simulink model "simulation model"  (R2022b)
settings: Solver=VariableStepAuto  StartTime=0.0  StopTime=2  RelTol=1e-3
undefined symbols (not defined in the file): a_prop, ACCtime, alfa, alfaPRO, Ba, Bf, Bp, Bv, IPR, matrixA, Ng_safe, No_perf, No_safe, Np, Np_safe, optimal_rotation, P3tDIVP2t_perf, P3tDIVP2t_safe, Q, Q_safe, T45_perf, T45_safe, Wf, xfuel, xlin, y, Yangle
libraries: fl_lib x31, nesl_utility x15, sh_lib x14, simulink x7, slpidlib x4, SimscapeFluids_lib x3
(part 1 of 2)
settings Model: PacingRate=10  Creator=48519  LastModifiedBy=48519
settings ModelReferenceCC: EnableRefExpFcnMdlSchedulingChecks=on

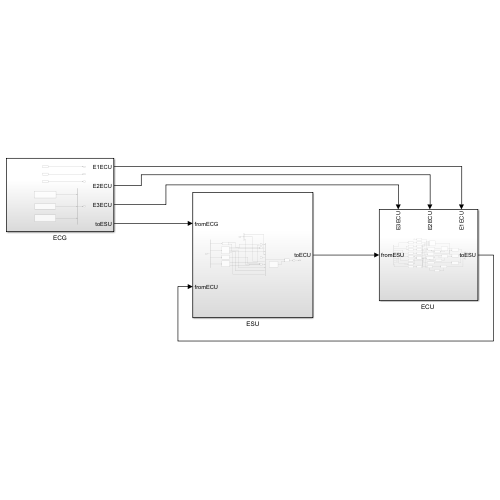
[thumbnail: Simulink's stored preview of the top-level diagram]
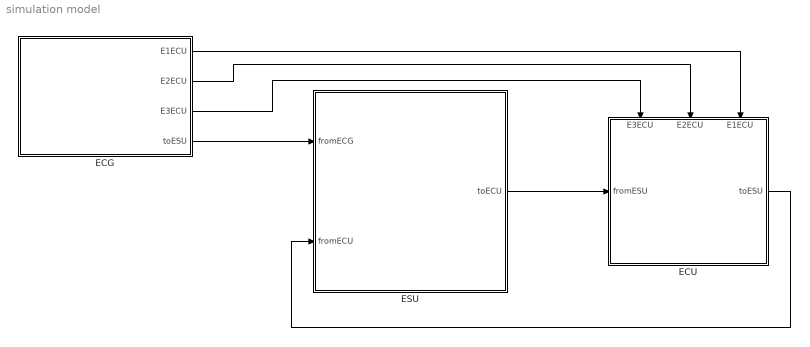
== system simulation model ==
  ECG : Subsystem
  "ECU " : Subsystem
      settings: PortSchema="{\"entries\":[{\"content\":{\"sides\":[{\"content\":{\"connectorIds\":[\"In1\"]},\"type\":\"ConnectorPlacement.EquallySpacedRectSide\",\"uuid\":\"8033a1fc-fa43-4d06-87e8-a4fef786c523\"},{\"content\":{\"connectorIds\":[\"Out1\"],\"side\":\"RIGHT\"},\"type\":\"ConnectorPlacement.EquallySpacedRectSide\",\"uuid\":\"5ca676c1-3d8d-4463-b14b-f5be12773dca\"},{\"content\":{\"connectorIds\":[\"In2\",\"In3\",\"In4\"],\"side\":\"TOP\"},\"type\":\"ConnectorPlacement.EquallySpacedRectSide\",\"uuid\":\"b18e2333-642d-4289-9df9-5f2a20e0ab9d\"}]},\"type\":\"ConnectorPlacement.EquallySpacedConnector\",\"uuid\":\"ecce7f03-20fc-4eea-af2c-957349ea8142\"}],\"packageUris\":[\"http://schema.mathworks.com/mf0/Connector/R2020b\"],\"version\":\"1.0\"}"
  ESU : Subsystem
  wires:
  ECG/4(toESU) -> ESU/1(fromECG)
  ESU/1(toECU) -> "ECU "/1(fromESU)
  "ECU "/1(toESU) -> ESU/2(fromECU)
  ECG/3(E3ECU) -> "ECU "/2(E3ECU)
  ECG/2(E2ECU) -> "ECU "/3(E2ECU)
  ECG/1(E1ECU) -> "ECU "/4(E1ECU)

== system simulation model/ECG ==
  Bus Creator : BusCreator  Inputs=4
  Emergency4 : Subsystem
  Emergency5 : Subsystem
  Emergency6 : Subsystem
  From Workspace : FromWorkspace  VariableName=Emerg3
  From Workspace1 : FromWorkspace  VariableName=Emerg1
  From Workspace2 : FromWorkspace  VariableName=Emerg2
  E1ECU : Outport
  E2ECU : Outport  Port=2
  E3ECU : Outport  Port=3
  toESU : Outport  Port=4
  wires:
  Emergency6/1(dP3e6) -> Bus Creator/4
  From Workspace1/1 -> E1ECU/1
  From Workspace/1 -> E3ECU/1
  From Workspace2/1 -> E2ECU/1
  Emergency4/1(dP2e4) -> Bus Creator/1
  Emergency5/2(dT1e5) -> Bus Creator/3
  Emergency5/1(dP0e5) -> Bus Creator/2
  Bus Creator/1 -> toESU/1

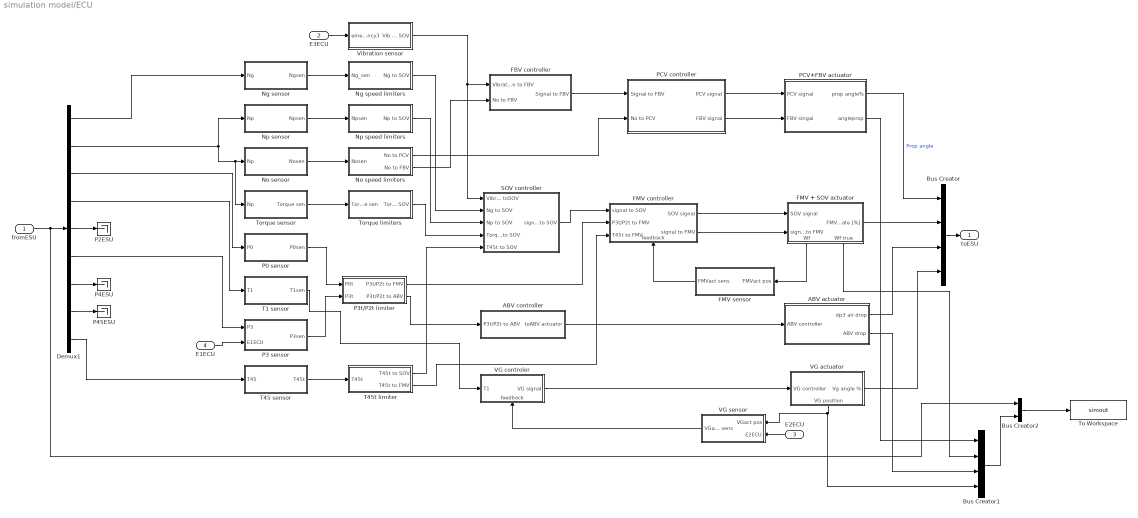
== system simulation model/ECU  ==
  fromESU : Inport
  E3ECU : Inport  Port=2
  E2ECU : Inport  Port=3
  E1ECU : Inport  Port=4
  " FMV controller" : Subsystem
      settings: PortSchema="{\"entries\":[{\"content\":{\"sides\":[{\"content\":{\"connectorIds\":[\"In1\",\"In2\",\"In3\"]},\"type\":\"ConnectorPlacement.EquallySpacedRectSide\",\"uuid\":\"38a2bfe9-8c47-42f1-bcd8-9832b9b327c4\"},{\"content\":{\"connectorIds\":[\"Out1\",\"Out2\"],\"side\":\"RIGHT\"},\"type\":\"ConnectorPlacement.EquallySpacedRectSide\",\"uuid\":\"0c090e16-2748-47be-b0e4-e5bed405b7d9\"},{\"content\":{\"connectorIds\":[],\"side\":\"TOP\"},\"type\":\"ConnectorPlacement.EquallySpacedRectSide\",\"uuid\":\"289f8d23-a454-4bfb-b029-d000a7415460\"},{\"content\":{\"connectorIds\":[\"In4\"],\"side\":\"BOTTOM\"},\"type\":\"ConnectorPlacement.EquallySpacedRectSide\",\"uuid\":\"f8021000-ba0a-47f6-928e-a2ead77e7ac1\"}]},\"type\":\"ConnectorPlacement.EquallySpacedConnector\",\"uuid\":\"1bac82f5-ade2-4038-9fa3-c74e21ed34d4\"}],\"packageUris\":[\"http://schema.mathworks.com/mf0/Connector/R2020b\"],\"version\":\"1.0\"}"
  ABV actuator : Subsystem
  ABV controller : Subsystem
  Bus Creator : BusCreator  Inputs=4
  Bus Creator1 : BusCreator  Inputs=4
  Bus Creator2 : BusCreator  Inputs=2
  Demux1 : Demux  Outputs=9
  FBV controller : Subsystem
  FMV + SOV actuator : Subsystem
      settings: PortSchema="{\"entries\":[{\"content\":{\"sides\":[{\"content\":{\"connectorIds\":[\"In1\",\"In2\"]},\"type\":\"ConnectorPlacement.EquallySpacedRectSide\",\"uuid\":\"38a2bfe9-8c47-42f1-bcd8-9832b9b327c4\"},{\"content\":{\"connectorIds\":[\"Out1\"],\"side\":\"RIGHT\"},\"type\":\"ConnectorPlacement.EquallySpacedRectSide\",\"uuid\":\"0c090e16-2748-47be-b0e4-e5bed405b7d9\"},{\"content\":{\"connectorIds\":[],\"side\":\"TOP\"},\"type\":\"ConnectorPlacement.EquallySpacedRectSide\",\"uuid\":\"289f8d23-a454-4bfb-b029-d000a7415460\"},{\"content\":{\"connectorIds\":[\"Out2\",\"Out3\"],\"side\":\"BOTTOM\"},\"type\":\"ConnectorPlacement.EquallySpacedRectSide\",\"uuid\":\"e366b5da-b3ec-4e5d-b0ef-8b87cef1eb6e\"}]},\"type\":\"ConnectorPlacement.EquallySpacedConnector\",\"uuid\":\"1bac82f5-ade2-4038-9fa3-c74e21ed34d4\"}],\"packageUris\":[\"http://schema.mathworks.com/mf0/Connector/R2020b\"],\"version\":\"1.0\"}"
  FMV sensor : Subsystem
  Ng sensor : Subsystem
  Ng speed limiters : Subsystem
  No sensor : Subsystem
  No speed limiters : Subsystem
  Np sensor : Subsystem
  Np speed limiters : Subsystem
  P0 sensor : Subsystem
  P2ESU : Terminator
  P3 sensor : Subsystem
  P3t/P2t limiter : Subsystem
  P45ESU : Terminator
  P4ESU : Terminator
  PCV controller : Subsystem
  PCV+FBV actuator : Subsystem
  SOV controller : Subsystem
  T1 sensor : Subsystem
  T45 sensor : Subsystem
  T45t limiter : Subsystem
  To Workspace : ToWorkspace  VariableName=simout  SaveFormat=Timeseries  SampleTime=-1
  Torque limiters : Subsystem
  Torque sensor : Subsystem
  VG actuator : Subsystem
      settings: PortSchema="{\"entries\":[{\"content\":{\"sides\":[{\"content\":{\"connectorIds\":[\"In1\"]},\"type\":\"ConnectorPlacement.EquallySpacedRectSide\",\"uuid\":\"39b00fd1-fd74-4dff-8589-67b80ee9d21f\"},{\"content\":{\"connectorIds\":[\"Out1\"],\"side\":\"RIGHT\"},\"type\":\"ConnectorPlacement.EquallySpacedRectSide\",\"uuid\":\"03fd2ba7-5317-42ec-98e7-2911bf7d9f9e\"},{\"content\":{\"connectorIds\":[],\"side\":\"TOP\"},\"type\":\"ConnectorPlacement.EquallySpacedRectSide\",\"uuid\":\"f7078396-c4bb-405d-aad9-135faa07c4e1\"},{\"content\":{\"connectorIds\":[\"Out2\"],\"side\":\"BOTTOM\"},\"type\":\"ConnectorPlacement.EquallySpacedRectSide\",\"uuid\":\"db5e57f9-c653-4944-8a82-ef51bf9c1c7f\"}]},\"type\":\"ConnectorPlacement.EquallySpacedConnector\",\"uuid\":\"a5cbbca1-7c96-4ab0-8754-d29e08537f1a\"}],\"packageUris\":[\"http://schema.mathworks.com/mf0/Connector/R2020b\"],\"version\":\"1.0\"}"
  VG controler : Subsystem
      settings: PortSchema="{\"entries\":[{\"content\":{\"sides\":[{\"content\":{\"connectorIds\":[\"In1\"]},\"type\":\"ConnectorPlacement.EquallySpacedRectSide\",\"uuid\":\"38a2bfe9-8c47-42f1-bcd8-9832b9b327c4\"},{\"content\":{\"connectorIds\":[\"Out1\"],\"side\":\"RIGHT\"},\"type\":\"ConnectorPlacement.EquallySpacedRectSide\",\"uuid\":\"0c090e16-2748-47be-b0e4-e5bed405b7d9\"},{\"content\":{\"connectorIds\":[],\"side\":\"TOP\"},\"type\":\"ConnectorPlacement.EquallySpacedRectSide\",\"uuid\":\"289f8d23-a454-4bfb-b029-d000a7415460\"},{\"content\":{\"connectorIds\":[\"In2\"],\"side\":\"BOTTOM\"},\"type\":\"ConnectorPlacement.EquallySpacedRectSide\",\"uuid\":\"9fd355d9-d690-4719-8550-140a79b88711\"}]},\"type\":\"ConnectorPlacement.EquallySpacedConnector\",\"uuid\":\"1bac82f5-ade2-4038-9fa3-c74e21ed34d4\"}],\"packageUris\":[\"http://schema.mathworks.com/mf0/Connector/R2020b\"],\"version\":\"1.0\"}"
  VG sensor : Subsystem
  Vibration sensor : Subsystem
  toESU : Outport
  wires:
  Ng sensor/1(Ngsen) -> Ng speed limiters/1(Ng_sen)
  Demux1/1 -> Ng sensor/1(Ng)
  Demux1/2 -> Np sensor/1(Np), Torque sensor/1(Np), No sensor/1(Np)
  fromESU/1 -> Bus Creator2/1, Demux1/1
  Demux1/3 -> P0 sensor/1(P0)
  Demux1/4 -> T1 sensor/1(T1)
  Demux1/5 -> P2ESU/1
  Demux1/6 -> P3 sensor/1(P3)
  Demux1/7 -> P4ESU/1
  Demux1/8 -> P45ESU/1
  Demux1/9 -> T45 sensor/1(T45)
  Np sensor/1(Npsen) -> Np speed limiters/1(Npsen)
  No sensor/1(Nosen) -> No speed limiters/1(Nosen)
  Torque sensor/1(Torque sen) -> Torque limiters/1(Torque sen)
  P3 sensor/1(P3sen) -> P3t/P2t limiter/2(P3t)
  P0 sensor/1(P0sen) -> P3t/P2t limiter/1(P0t)
  T45 sensor/1(T45t) -> T45t limiter/1(T45t)
  T45t limiter/2(T45t to FMV) -> " FMV controller"/3(T45t to FMV)
  P3t/P2t limiter/1(P3t/P2t to FMV) -> " FMV controller"/2(P3t/P2t to FMV)
  Ng speed limiters/1(Ng to SOV) -> SOV controller/2(Ng to SOV)
  Np speed limiters/1(Np to SOV) -> SOV controller/3(Np to SOV)
  " FMV controller"/2(signal to FMV) -> FMV + SOV actuator/2(signal to FMV)
  No speed limiters/1(No to PCV) -> PCV controller/2(No to PCV)
  No speed limiters/2(No to FBV) -> FBV controller/2(No to FBV)
  PCV controller/1(PCV signal) -> PCV+FBV actuator/1(PCV signal)
  Vibration sensor/1(Vib to SOV) -> FBV controller/1(Vibration to FBV), SOV controller/1(Vibration toSOV)
  T45t limiter/1(T45t to SOV) -> SOV controller/5(T45t to SOV)
  P3t/P2t limiter/2(P3t/P2t to ABV) -> ABV controller/1(P3t/P2t to ABV)
  PCV+FBV actuator/1(prop angle%) -> Bus Creator/1  "Prop angle"
  FMV + SOV actuator/1(FMV flow rate [%]) -> Bus Creator/2
  ABV actuator/1(dp3 air drop) -> Bus Creator/3
  VG actuator/1(Vg angle %) -> Bus Creator/4
  Bus Creator/1 -> toESU/1
  Torque limiters/1(Torque to SOV) -> SOV controller/4(Torque to SOV)
  E3ECU/1 -> Vibration sensor/1(emergency3)
  E1ECU/1 -> P3 sensor/2(E1ECU)
  E2ECU/1 -> VG sensor/2(E2ECU)
  FMV + SOV actuator/2(Wf) -> FMV sensor/1(FMVact pos)
  FMV sensor/1(FMVact sens) -> " FMV controller"/4(feedback)
  VG actuator/2(VG position) -> Bus Creator1/4, VG sensor/1(VGact pos)
  VG sensor/1(VGact sens) -> VG controler/2(feedback)
  PCV controller/2(FBV signal) -> PCV+FBV actuator/2(FBV singal)
  " FMV controller"/1(SOV signal) -> FMV + SOV actuator/1(SOV signal)
  T1 sensor/1(T1sen) -> VG controler/1(T1)
  Bus Creator1/1 -> Bus Creator2/2
  ABV actuator/2(ABV drop) -> Bus Creator1/3
  FMV + SOV actuator/3(Wf true) -> Bus Creator1/2
  PCV+FBV actuator/2(angleprop) -> Bus Creator1/1
  Bus Creator2/1 -> To Workspace/1
  FBV controller/1(Signal to FBV) -> PCV controller/1(Signal to FBV)
  SOV controller/1(signal to SOV) -> " FMV controller"/1(signal to SOV)
  ABV controller/1(toABV actuator) -> ABV actuator/1(ABV controller)
  VG controler/1(VG signal) -> VG actuator/1(VG controller)

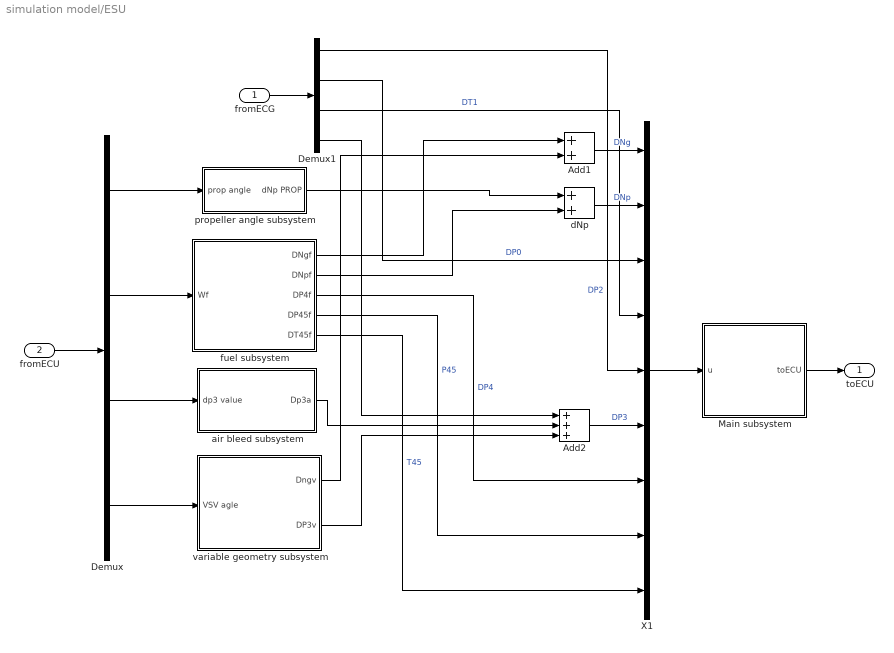
== system simulation model/ESU ==
  fromECG : Inport
  fromECU : Inport  Port=2
  Add1 : Sum
  Add2 : Sum  Inputs=+++
  Demux : Demux
  Demux1 : Demux
  Main subsystem : Subsystem
  X1 : BusCreator  Inputs=9
  air bleed subsystem : Subsystem
  dNp : Sum
  fuel subsystem : Subsystem
  propeller angle subsystem : Subsystem
  variable geometry subsystem : Subsystem
  toECU : Outport
  wires:
  fuel subsystem/2(DNpf) -> dNp/2
  fuel subsystem/3(DP4f) -> X1/7  "DP4"
  fuel subsystem/4(DP45f) -> X1/8  "P45"
  air bleed subsystem/1(Dp3a) -> Add2/2
  Demux/1 -> propeller angle subsystem/1(prop angle)
  Demux/4 -> variable geometry subsystem/1("VSV agle ")
  dNp/1 -> X1/2  "DNp"
  propeller angle subsystem/1(dNp PROP) -> dNp/1
  Add1/1 -> X1/1  "DNg"
  fuel subsystem/1(DNgf) -> Add1/1
  variable geometry subsystem/1(Dngv) -> Add1/2
  Demux1/1 -> X1/5  "DP2"
  Demux1/2 -> X1/3  "DP0"
  variable geometry subsystem/2(DP3v) -> Add2/3
  Add2/1 -> X1/6  "DP3"
  fuel subsystem/5(DT45f) -> X1/9  "T45"
  Demux1/3 -> X1/4  "DT1"
  Demux1/4 -> Add2/1
  X1/1 -> Main subsystem/1(u)
  Main subsystem/1(toECU) -> toECU/1
  fromECU/1 -> Demux/1
  Demux/3 -> air bleed subsystem/1(dp3 value)
  Demux/2 -> fuel subsystem/1(Wf)
  fromECG/1 -> Demux1/1

== system simulation model/ECG/Emergency4 ==
  Clock : Clock
  Clock1 : Clock
  Constant : Constant  Value=0
  Constant1 : Constant  Value=0
  From Workspace : FromWorkspace  VariableName=Emerg4
  Ramp : simulink/Sources/Ramp  slope=-0.07/450  start=ACCtime  InitialOutput=0
  Ramp1 : simulink/Sources/Ramp  slope=0.07/50  start=ACCtime+30  InitialOutput=0
  Switch : Switch  Criteria=u2 > Threshold  Threshold=ACCtime+40  SaturateOnIntegerOverflow=off  InputSameDT=off
  Switch1 : Switch  Criteria=u2 > Threshold  Threshold=ACCtime+30  SaturateOnIntegerOverflow=off  InputSameDT=off
  Switch2 : Switch  Criteria=u2 > Threshold  SaturateOnIntegerOverflow=off  InputSameDT=off
  dP2e4 : Outport
  wires:
  Ramp1/1 -> Switch1/1
  Ramp/1 -> Switch1/3
  Switch1/1 -> Switch/3
  Constant/1 -> Switch/1
  Clock/1 -> Switch/2
  Clock1/1 -> Switch1/2
  From Workspace/1 -> Switch2/2
  Constant1/1 -> Switch2/3
  Switch/1 -> Switch2/1
  Switch2/1 -> dP2e4/1

== system simulation model/ECG/Emergency5 ==
  Clock3 : Clock
  Constant1 : Constant  Value=0
  Constant2 : Constant  Value=0
  From Workspace : FromWorkspace  VariableName=Emerg5
  Ramp2 : simulink/Sources/Ramp  slope=-(0.05)/(300*300/2)  start=ACCtime  InitialOutput=0
  Switch2 : Switch  Criteria=u2 > Threshold  SaturateOnIntegerOverflow=off  InputSameDT=off
  Switch3 : Switch  Criteria=u2 > Threshold  Threshold=ACCtime+300  SaturateOnIntegerOverflow=off  InputSameDT=off
  dP0e5 : Outport
  dT1e5 : Outport  Port=2
  wires:
  Switch2/1 -> dT1e5/1, dP0e5/1
  Constant2/1 -> Switch3/1
  Ramp2/1 -> Switch3/3
  Clock3/1 -> Switch3/2
  Constant1/1 -> Switch2/3
  From Workspace/1 -> Switch2/2
  Switch3/1 -> Switch2/1

== system simulation model/ECG/Emergency6 ==
  Clock2 : Clock
  Constant1 : Constant  Value=0
  Constant2 : Constant  Value=0
  From Workspace : FromWorkspace  VariableName=Emerg6
  Ramp3 : simulink/Sources/Ramp  slope=-0.6/25  start=ACCtime  InitialOutput=0
  Switch1 : Switch  Criteria=u2 > Threshold  SaturateOnIntegerOverflow=off  InputSameDT=off
  Switch2 : Switch  Criteria=u2 > Threshold  Threshold=ACCtime+5  SaturateOnIntegerOverflow=off  InputSameDT=off
  dP3e6 : Outport
  wires:
  Ramp3/1 -> Switch2/3
  Constant1/1 -> Switch2/1
  Clock2/1 -> Switch2/2
  From Workspace/1 -> Switch1/2
  Constant2/1 -> Switch1/3
  Switch2/1 -> Switch1/1
  Switch1/1 -> dP3e6/1

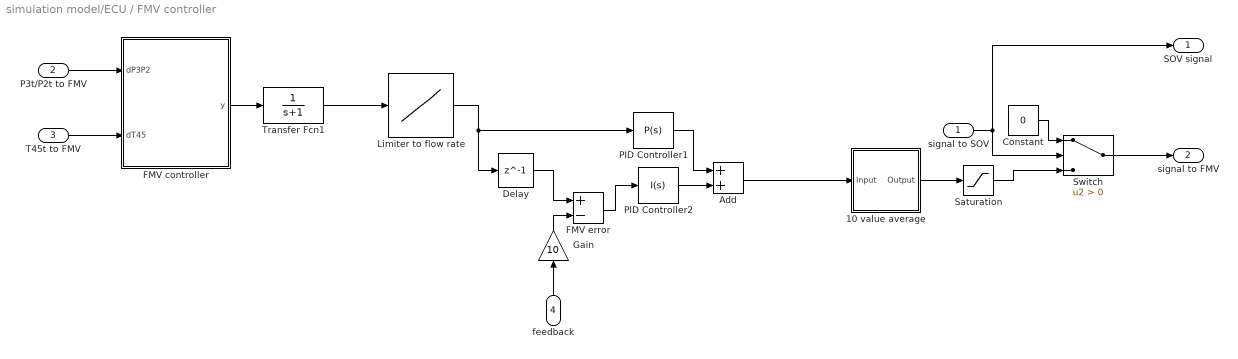
== system simulation model/ECU / FMV controller ==
  signal to SOV : Inport
  P3t/P2t to FMV : Inport  Port=2
  T45t to FMV : Inport  Port=3
  feedback : Inport  Port=4
  10 value average : Subsystem
  Add : Sum
  Constant : Constant  Value=0
  Delay : Delay  DelayLength=1  SampleTime=0.01
  FMV controller : MATLAB Function  TreatAsAtomicUnit=on
  FMV error : Sum  Inputs=+-
  Gain : Gain  Gain=10
  Limiter to flow rate : Lookup_n-D  NumberOfTableDimensions=1  BreakpointsForDimension1=xfuel  Table=Wf  InternalRulePriority=Speed  RndMeth=Simplest
  PID Controller1 : slpidlib/PID Controller  Controller=P  Form=Parallel  TimeDomain=Continuous-time  UseExternalTs=off  SampleTime=-1  IntegratorMethod=Forward Euler  FilterMethod=Forward Euler  ControllerParametersSource=internal  P=11.8694/0.44  I=0  UseKiTs=off  D=0  N=100  UseFilter=on  TunerSelectOption=Transfer Function Based (PID Tuner App)  InitialConditionSource=internal  InitialConditionForIntegrator=0  InitialConditionForFilter=0  DifferentiatorICPrevScaledInput=0  ExternalReset=none  TrackingMode=off  Kt=1  LimitOutput=off  SatLimitsSource=internal  UpperSaturationLimit=inf  LowerSaturationLimit=-inf  LinearizeAsGain=on  AntiWindupMode=none  Kb=1  LimitIntegrator=off  UpperIntegratorSaturationLimit=inf  LowerIntegratorSaturationLimit=-inf  POutMin=[]  POutMax=[]  IOutMin=[]  IOutMax=[]  DOutMin=[]  DOutMax=[]  NOutMin=[]  NOutMax=[]  SumOutMin=[]  SumOutMax=[]  SaturationOutMin=[]  SaturationOutMax=[]  PParamMin=[]  PParamMax=[]  IParamMin=[]  IParamMax=[]  DParamMin=[]  DParamMax=[]  NParamMin=[]  NParamMax=[]  KbParamMin=[]  KbParamMax=[]  KtParamMin=[]  KtParamMax=[]  KbOutMin=[]  KbOutMax=[]  KtOutMin=[]  KtOutMax=[]  IntegratorOutMin=[]  IntegratorOutMax=[]  FilterOutMin=[]  FilterOutMax=[]  SumI1OutMin=[]  SumI1OutMax=[]  SumI2OutMin=[]  SumI2OutMax=[]  SumI3OutMin=[]  SumI3OutMax=[]  SumI4OutMin=[]  SumI4OutMax=[]  SumDOutMin=[]  SumDOutMax=[]  DifferentiatorOutMin=[]  DifferentiatorOutMax=[]  FilterDiffOutCoefMin=[]  FilterDiffOutCoefMax=[]  ReciprocalOutMin=[]  ReciprocalOutMax=[]  SumDenOutMin=[]  SumDenOutMax=[]  SumNumOutMin=[]  SumNumOutMax=[]  DivideOutMin=[]  DivideOutMax=[]  UdiffTsProdOutMin=[]  UdiffTsProdOutMax=[]  NTsProdOutMin=[]  NTsProdOutMax=[]  UintegralTsProdOutMin=[]  UintegralTsProdOutMax=[]  UngainTsProdOutMin=[]  UngainTsProdOutMax=[]  ClampingZeroOutDataTypeStr=Inherit: Inherit via back propagation  ClampingZeroOutMin=[]  ClampingZeroOutMax=[]  FilterDenConstantOutDataTypeStr=Inherit: Inherit via back propagation  FilterDenConstantOutMin=[]  FilterDenConstantOutMax=[]  PCopyOutDataTypeStr=Inherit: Inherit via back propagation  PCopyOutMin=[]  PCopyOutMax=[]  NCopyOutDataTypeStr=Inherit: Inherit via back propagation  NCopyOutMin=[]  NCopyOutMax=[]  IntegratorContinuousStateAttributes=''  IntegratorStateMustResolveToSignalObject=off  IntegratorRTWStateStorageClass=Auto  FilterContinuousStateAttributes=''  FilterStateMustResolveToSignalObject=off  FilterRTWStateStorageClass=Auto  ParallelPVariant=InternalParameters  IdealPVariant=Disabled  IVariant=Disabled  DVariant=Disabled  IntegratorVariant=Disabled  SatVariant=Disabled  AWVariant=Disabled  PCopyVariant=Disabled  TRVariant=Disabled  FdbkBlocksVariant=Forward  IdealPFdbkVariant=Disabled  SatFdbkVariant=Disabled  DerivativeFilterVariant=Disabled  NVariant=Disabled  NCopyVariant=Disabled_SignalSpec  FilterICVariant=Disabled  IntegratorICVariant=Disabled  ExternalResetVariant=Disabled  TRSumVariant=Passthrough  SumFdbkVariant=Disabled  SumVariant=Passthrough_P  TsampFilterVariant=InternalTs  TsampNgainVariant=Passthrough  TsampIntegralVariant=Disabled_SignalSpec  ExternalSaturationOutDataTypeStr=Inherit: Same as second input
  PID Controller2 : slpidlib/PID Controller  Controller=I  Form=Parallel  TimeDomain=Continuous-time  UseExternalTs=off  SampleTime=-1  IntegratorMethod=Forward Euler  FilterMethod=Forward Euler  ControllerParametersSource=internal  P=1  I=0  UseKiTs=off  D=0  N=100  UseFilter=on  TunerSelectOption=Transfer Function Based (PID Tuner App)  InitialConditionSource=internal  InitialConditionForIntegrator=0  InitialConditionForFilter=0  DifferentiatorICPrevScaledInput=0  ExternalReset=none  TrackingMode=off  Kt=1  LimitOutput=on  SatLimitsSource=internal  UpperSaturationLimit=inf  LowerSaturationLimit=-inf  LinearizeAsGain=on  AntiWindupMode=clamping  Kb=1  LimitIntegrator=on  UpperIntegratorSaturationLimit=10  LowerIntegratorSaturationLimit=-10  POutMin=[]  POutMax=[]  IOutMin=[]  IOutMax=[]  DOutMin=[]  DOutMax=[]  NOutMin=[]  NOutMax=[]  SumOutMin=[]  SumOutMax=[]  SaturationOutMin=[]  SaturationOutMax=[]  PParamMin=[]  PParamMax=[]  IParamMin=[]  IParamMax=[]  DParamMin=[]  DParamMax=[]  NParamMin=[]  NParamMax=[]  KbParamMin=[]  KbParamMax=[]  KtParamMin=[]  KtParamMax=[]  KbOutMin=[]  KbOutMax=[]  KtOutMin=[]  KtOutMax=[]  IntegratorOutMin=[]  IntegratorOutMax=[]  FilterOutMin=[]  FilterOutMax=[]  SumI1OutMin=[]  SumI1OutMax=[]  SumI2OutMin=[]  SumI2OutMax=[]  SumI3OutMin=[]  SumI3OutMax=[]  SumI4OutMin=[]  SumI4OutMax=[]  SumDOutMin=[]  SumDOutMax=[]  DifferentiatorOutMin=[]  DifferentiatorOutMax=[]  FilterDiffOutCoefMin=[]  FilterDiffOutCoefMax=[]  ReciprocalOutMin=[]  ReciprocalOutMax=[]  SumDenOutMin=[]  SumDenOutMax=[]  SumNumOutMin=[]  SumNumOutMax=[]  DivideOutMin=[]  DivideOutMax=[]  UdiffTsProdOutMin=[]  UdiffTsProdOutMax=[]  NTsProdOutMin=[]  NTsProdOutMax=[]  UintegralTsProdOutMin=[]  UintegralTsProdOutMax=[]  UngainTsProdOutMin=[]  UngainTsProdOutMax=[]  ClampingZeroOutDataTypeStr=Inherit: Inherit via back propagation  ClampingZeroOutMin=[]  ClampingZeroOutMax=[]  FilterDenConstantOutDataTypeStr=Inherit: Inherit via back propagation  FilterDenConstantOutMin=[]  FilterDenConstantOutMax=[]  PCopyOutDataTypeStr=Inherit: Inherit via back propagation  PCopyOutMin=[]  PCopyOutMax=[]  NCopyOutDataTypeStr=Inherit: Inherit via back propagation  NCopyOutMin=[]  NCopyOutMax=[]  IntegratorContinuousStateAttributes=''  IntegratorStateMustResolveToSignalObject=off  IntegratorRTWStateStorageClass=Auto  FilterContinuousStateAttributes=''  FilterStateMustResolveToSignalObject=off  FilterRTWStateStorageClass=Auto  ParallelPVariant=Disabled  IdealPVariant=Disabled  IVariant=InternalParameters  DVariant=Disabled  IntegratorVariant=Continuous  SatVariant=Enabled  AWVariant=ContClampingParallel  PCopyVariant=Disabled  TRVariant=Disabled  FdbkBlocksVariant=Forward  IdealPFdbkVariant=Disabled  SatFdbkVariant=Disabled  DerivativeFilterVariant=Disabled  NVariant=Disabled  NCopyVariant=Disabled_SignalSpec  FilterICVariant=Disabled  IntegratorICVariant=InternalICs  ExternalResetVariant=Disabled  TRSumVariant=Passthrough  SumFdbkVariant=Disabled  SumVariant=Passthrough_I  TsampFilterVariant=InternalTs  TsampNgainVariant=Passthrough  TsampIntegralVariant=Passthrough  ExternalSaturationOutDataTypeStr=Inherit: Same as second input
  Saturation : Saturate  UpperLimit=11.8694*1.25  LowerLimit=11.8694*0.75
  Switch : Switch  Criteria=u2 > Threshold  SaturateOnIntegerOverflow=off  InputSameDT=off
  Transfer Fcn1 : TransferFcn  Denominator=[1 1]
  SOV signal : Outport
  signal to FMV : Outport  Port=2
  wires:
  Limiter to flow rate/1 -> PID Controller1/1, Delay/1
  P3t/P2t to FMV/1 -> FMV controller/1(dP3P2)
  T45t to FMV/1 -> FMV controller/2(dT45)
  FMV controller/1(y) -> Transfer Fcn1/1
  Switch/1 -> signal to FMV/1
  Constant/1 -> Switch/1
  FMV error/1 -> PID Controller2/1
  PID Controller1/1 -> Add/1
  PID Controller2/1 -> Add/2
  Add/1 -> 10 value average/1(Input)
  Saturation/1 -> Switch/3
  signal to SOV/1 -> SOV signal/1, Switch/2
  feedback/1 -> Gain/1
  10 value average/1(Output) -> Saturation/1
  Gain/1 -> FMV error/2
  Delay/1 -> FMV error/1
  Transfer Fcn1/1 -> Limiter to flow rate/1

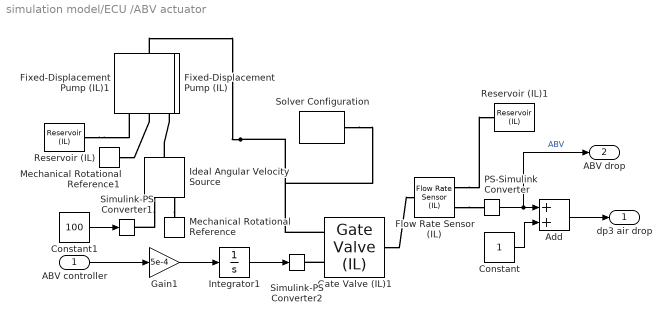
== system simulation model/ECU /ABV actuator ==
  ABV controller : Inport
  Add : Sum
  Constant : Constant
  Constant1 : Constant  Value=100
  Fixed-Displacement Pump (IL) : SimscapeFluids_lib/Isothermal Liquid/Pumps & Motors/Fixed-Displacement Pump (IL)  leakage_friction_spec=fluids.isothermal_liquid.pumps_motors.enum.pump_motor_loss_spec.analytical  displacement=30 cm^3/rev  omega_nominal=188 rad/s  p_nominal=10 MPa  vol_eff_nominal=0.92  mech_eff_nominal=0.88  no_load_torque=0 N*m  p_diff_eff_TLU=[.1, 1, 2] MPa  omega_eff_TLU=[25, 50, 100, 200, 300, 400] rad/s  vol_eff_TLU=[.816, .908, .954, .977, .981, .984; .325, .663, .831, .916, .925, .946; .137, .568, .78, .892, .893, .91]  mech_eff_TLU=[.996, .996, .996, .996, .996, .996; .988, .989, .989, .989, .989, .99; .981, .981, .982, .982, .983, .984]  p_diff_loss_TLU=[.1, 1, 2] MPa  omega_loss_TLU=[25, 50, 100, 200, 300, 400] rad/s  vol_loss_TLU=1e-3 * [.023, .023, .023, .023, .0285, .032; .0844, .0842, .0845, .084, .1125, .108; .1079, .108, .11, .108, .1605, .18] m^3/s  mech_loss_TLU=[.002, .002, .002, .002, .002, .002; .0607, .0556, .0556, .0556, .0556, .0505; .1937, .1937, .1833, .1833, .1729, .1626] N*m  vol_eff_min=1e-3  vol_eff_max=1  mech_eff_min=1e-3  mech_eff_max=1  pressure_threshold=1e-3 MPa  omega_threshold=10 rad/s  quadrant_check=simscape.enum.assert.action.none  pump_mode_check=simscape.enum.assert.action.none  pressure_check=simscape.enum.assert.action.none  p_min_valid=0.101325 MPa
      settings: LogSimulationData=on  InternalSimscapePortConfiguration="{\"Bottom\":[{\"id\":\"A\",\"label\":\"A\",\"type\":\"foundation.isothermal_liquid.isothermal_liquid\"}],\"Left\":[],\"Right\":[{\"id\":\"R\",\"label\":\"R\",\"type\":\"foundation.mechanical.rotational.rotational\"},{\"id\":\"C\",\"label\":\"C\",\"type\":\"foundation.mechanical.rotational.rotational\"}],\"Top\":[{\"id\":\"B\",\"label\":\"B\",\"type\":\"foundation.isothermal_liquid.isothermal_liquid\"}]}"
  Fixed-Displacement Pump (IL)1 : SimscapeFluids_lib/Isothermal Liquid/Pumps & Motors/Fixed-Displacement Pump (IL)  leakage_friction_spec=fluids.isothermal_liquid.pumps_motors.enum.pump_motor_loss_spec.analytical  displacement=30 cm^3/rev  omega_nominal=188 rad/s  p_nominal=10 MPa  vol_eff_nominal=0.92  mech_eff_nominal=0.88  no_load_torque=0 N*m  p_diff_eff_TLU=[.1, 1, 2] MPa  omega_eff_TLU=[25, 50, 100, 200, 300, 400] rad/s  vol_eff_TLU=[.816, .908, .954, .977, .981, .984; .325, .663, .831, .916, .925, .946; .137, .568, .78, .892, .893, .91]  mech_eff_TLU=[.996, .996, .996, .996, .996, .996; .988, .989, .989, .989, .989, .99; .981, .981, .982, .982, .983, .984]  p_diff_loss_TLU=[.1, 1, 2] MPa  omega_loss_TLU=[25, 50, 100, 200, 300, 400] rad/s  vol_loss_TLU=1e-3 * [.023, .023, .023, .023, .0285, .032; .0844, .0842, .0845, .084, .1125, .108; .1079, .108, .11, .108, .1605, .18] m^3/s  mech_loss_TLU=[.002, .002, .002, .002, .002, .002; .0607, .0556, .0556, .0556, .0556, .0505; .1937, .1937, .1833, .1833, .1729, .1626] N*m  vol_eff_min=1e-3  vol_eff_max=1  mech_eff_min=1e-3  mech_eff_max=1  pressure_threshold=1e-3 MPa  omega_threshold=10 rad/s  quadrant_check=simscape.enum.assert.action.none  pump_mode_check=simscape.enum.assert.action.none  pressure_check=simscape.enum.assert.action.none  p_min_valid=0.101325 MPa
      settings: LogSimulationData=on  InternalSimscapePortConfiguration="{\"Bottom\":[{\"id\":\"A\",\"label\":\"A\",\"type\":\"foundation.isothermal_liquid.isothermal_liquid\"}],\"Left\":[],\"Right\":[{\"id\":\"R\",\"label\":\"R\",\"type\":\"foundation.mechanical.rotational.rotational\"},{\"id\":\"C\",\"label\":\"C\",\"type\":\"foundation.mechanical.rotational.rotational\"}],\"Top\":[{\"id\":\"B\",\"label\":\"B\",\"type\":\"foundation.isothermal_liquid.isothermal_liquid\"}]}"
  Flow Rate Sensor (IL) : fl_lib/Isothermal Liquid/Sensors/Flow Rate Sensor (IL)  sensor_type=foundation.enum.mass_volumetric_sensor.mass
      settings: InternalSimscapePortConfiguration="{\"Bottom\":[],\"Left\":[{\"id\":\"A\",\"label\":\"A\",\"type\":\"foundation.isothermal_liquid.isothermal_liquid\"}],\"Right\":[{\"id\":\"B\",\"label\":\"B\",\"type\":\"foundation.isothermal_liquid.isothermal_liquid\"},{\"id\":\"M\",\"label\":\"M\",\"type\":\"output\"}],\"Top\":[]}"
  Gain1 : Gain  Gain=5e-4
  Gate Valve (IL)1 : SimscapeFluids_lib/Isothermal Liquid/Valves & Orifices/Flow Control Valves/Gate Valve (IL)  diam_orifice=5.2e-4 m  S_min=0 m  area_leak=1e-100 m^2  area=inf m^2  Cd=0.64  Re_c=150  smoothing_factor=0.01  pressure_recovery=simscape.enum.onoff.off  mdot_A_specify=off  mdot_A_priority=None  mdot_A=0 kg/s  mdot_A_nominal_specify=off  mdot_A_nominal_unit=kg/s  mdot_A_nominal_value=1  mdot_B_specify=off  mdot_B_priority=None  mdot_B=0 kg/s  mdot_B_nominal_specify=off  mdot_B_nominal_unit=kg/s  mdot_B_nominal_value=1
      settings: InternalSimscapePortConfiguration="{\"Bottom\":[],\"Left\":[{\"id\":\"A\",\"label\":\"A\",\"type\":\"foundation.isothermal_liquid.isothermal_liquid\"},{\"id\":\"S\",\"label\":\"S\",\"type\":\"input\"}],\"Right\":[{\"id\":\"B\",\"label\":\"B\",\"type\":\"foundation.isothermal_liquid.isothermal_liquid\"}],\"Top\":[]}"
  Ideal Angular Velocity Source : fl_lib/Mechanical/Mechanical Sources/Ideal Angular Velocity Source
  Integrator1 : Integrator  LimitOutput=on  UpperSaturationLimit=1
  Mechanical Rotational Reference : fl_lib/Mechanical/Rotational Elements/Mechanical Rotational Reference
  Mechanical Rotational Reference1 : fl_lib/Mechanical/Rotational Elements/Mechanical Rotational Reference
  PS-Simulink Converter : nesl_utility/PS-Simulink Converter  PhysicalDomain=network_engine_domain  SubClassName=ps_output  LeftPortType=input  RightPortType=output  PseudoPeriodic=off  Frequencies=[]  VectorFormat=inherit  Unit=inherit  AffineConversion=off
  Reservoir (IL) : fl_lib/Isothermal Liquid/Elements/Reservoir (IL)  reservoir_type=foundation.enum.constant_controlled.constant  pressure_spec=foundation.enum.pressure_spec.atmospheric  reservoir_pressure=0.101325 MPa
  Reservoir (IL)1 : fl_lib/Isothermal Liquid/Elements/Reservoir (IL)  reservoir_type=foundation.enum.constant_controlled.constant  pressure_spec=foundation.enum.pressure_spec.atmospheric  reservoir_pressure=0.101325 MPa
  Simulink-PS Converter1 : nesl_utility/Simulink-PS Converter  PhysicalDomain=network_engine_domain  SubClassName=ps_input  LeftPortType=input  RightPortType=output  PseudoPeriodic=off  Frequencies=[]  NoiseDistribution=none  NoiseParameters=[]  Unit=1  AffineConversion=off  FilteringAndDerivatives=provide  SimscapeFilterOrder=1  InputFilterTimeConstant=0.001  UdotUserProvided=0
  Simulink-PS Converter2 : nesl_utility/Simulink-PS Converter  PhysicalDomain=network_engine_domain  SubClassName=ps_input  LeftPortType=input  RightPortType=output  PseudoPeriodic=off  Frequencies=[]  NoiseDistribution=none  NoiseParameters=[]  Unit=1  AffineConversion=off  FilteringAndDerivatives=provide  SimscapeFilterOrder=1  InputFilterTimeConstant=0.001  UdotUserProvided=0
  Solver Configuration : nesl_utility/Solver Configuration  PhysicalDomain=network_engine_domain  SubClassName=solver  LeftPortType=input  RightPortType=generic  Tones=[]  Harmonics=[]  SimulateNoise=off  Profile=off  UseLocalSampling=off  EnableSwitchedLinearOptims=on  FrequencyDomain=off  UseCCode=off  RelTol=0.001  AbsTol=0.001  MinStep=1e-09  ToWorkspace=off  RevertToSquareIcSolve=off  NumHomotopyIterations=100  PhasorMode=off  PhasorModeNumHarmonics=1  ConsistencySolver=NEWTON_XTOL_AFTER_FTOL  IndexReductionMethod=DerivativeReplacement  DoDC=off  ResidualTolerance=1e-09  ConsistencyTolSource=GLOBAL  ConsistencyAbsTol=0.001  ConsistencyRelTol=0.001  ConsistencyTolFactor=0.001  UseLocalSolver=off  LocalSolverChoice=NE_BACKWARD_EULER_ADVANCER  ResolveIndetEquations=on  FunctionEvalNumThread=1  LocalSolverSampleTime=0.001  DoFixedCost=off  MaxNonlinIter=3  MaxModeIter=2  ComputeImpulses=off  ImpulseIterations=2  LinearAlgebra=auto  LinearAlgebraNumThread=0  EquationFormulation=NE_TIME_EF  DelaysMemoryBudget=1024  AutomaticFiltering=on  FilteringTimeConstant=0.001  PartitionStorageMethod=AS_NEEDED  PartitionMemoryBudget=1024  PartitionMethod=ROBUST
  dp3 air drop : Outport
  ABV drop : Outport  Port=2
  wires:
  Integrator1/1 -> Simulink-PS Converter2/1
  Gain1/1 -> Integrator1/1
  Constant1/1 -> Simulink-PS Converter1/1
  ABV controller/1 -> Gain1/1
  PS-Simulink Converter/1 -> ABV drop/1, Add/1  "ABV"
  Constant/1 -> Add/2
  Add/1 -> dp3 air drop/1
  connections:
  Fixed-Displacement Pump (IL)/LConn1 -- Gate Valve (IL)1/LConn1 -- Solver Configuration/RConn1
  Ideal Angular Velocity Source/LConn1 -- Fixed-Displacement Pump (IL)/RConn1
  Ideal Angular Velocity Source/RConn1 -- Simulink-PS Converter1/RConn1
  Flow Rate Sensor (IL)/RConn1 -- Reservoir (IL)1/LConn1
  Reservoir (IL)/LConn1 -- Fixed-Displacement Pump (IL)/RConn3
  Ideal Angular Velocity Source/RConn2 -- Mechanical Rotational Reference/LConn1
  Flow Rate Sensor (IL)/RConn2 -- PS-Simulink Converter/LConn1
  Gate Valve (IL)1/LConn2 -- Simulink-PS Converter2/RConn1
  Mechanical Rotational Reference1/LConn1 -- Fixed-Displacement Pump (IL)/RConn2
  Gate Valve (IL)1/RConn1 -- Flow Rate Sensor (IL)/LConn1

== system simulation model/ECU /ABV controller ==
  P3t/P2t to ABV : Inport
  Latch max value : simulink/Math Operations/MinMax Running Resettable  Function=max  vinit=0.0
  NOT RESET : Constant  Value=0
  toABV actuator : Outport
  wires:
  P3t/P2t to ABV/1 -> Latch max value/1
  NOT RESET/1 -> Latch max value/2
  Latch max value/1 -> toABV actuator/1

== system simulation model/ECU /FBV controller ==
  Vibration to FBV : Inport
  No to FBV : Inport  Port=2
  Add : Sum  OutMax=[1]
  Constant : Constant
  Gain : Gain  Gain=-2
  Latch max value : simulink/Math Operations/MinMax Running Resettable  Function=max  vinit=0.0
  NOT RESET : Constant  Value=0
  Subtract : Sum
  max=1 : Saturate  UpperLimit=1  LowerLimit=0
  Signal to FBV : Outport
  wires:
  Add/1 -> max=1/1
  Vibration to FBV/1 -> Add/1
  No to FBV/1 -> Add/2
  NOT RESET/1 -> Latch max value/2
  max=1/1 -> Latch max value/1
  Subtract/1 -> Signal to FBV/1
  Latch max value/1 -> Gain/1
  Gain/1 -> Subtract/2
  Constant/1 -> Subtract/1

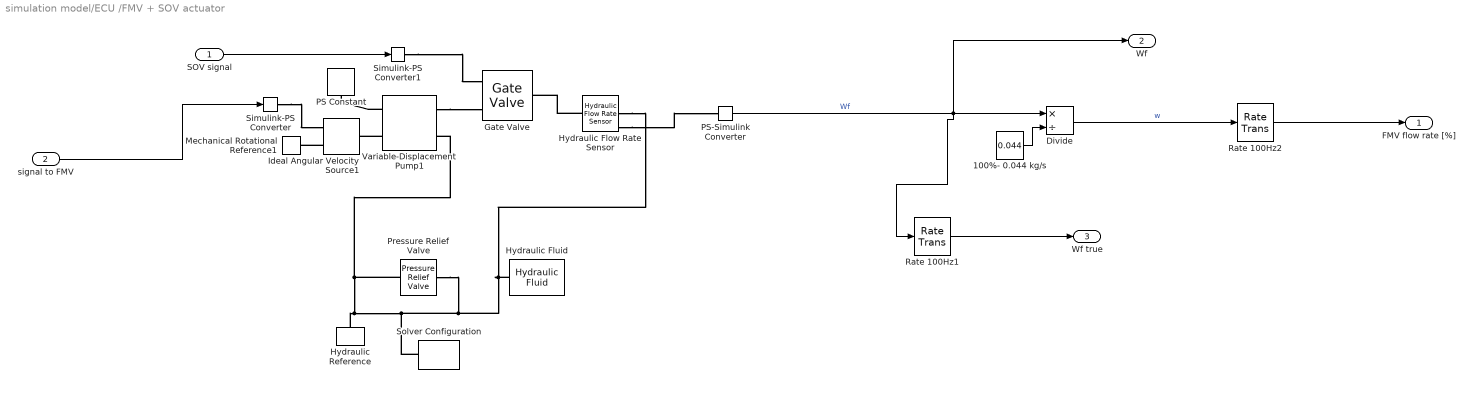
== system simulation model/ECU /FMV + SOV actuator ==
  SOV signal : Inport
  signal to FMV : Inport  Port=2
  100%- 0.044 kg/s : Constant  Value=0.044
  Divide : Product  Inputs=*/
  Gate Valve : sh_lib/Valves/Flow Control Valves/Gate Valve  d_gate=0.01 m  x_0=-0.1 m  C_d=10^12  A_leak=1e-12 m^2  lam_spec=1  B_lam=0.999  Re_cr=10
      settings: InternalSimscapePortConfiguration="{\"Bottom\":[],\"Left\":[{\"id\":\"S\",\"label\":\"S\",\"type\":\"input\"},{\"id\":\"A\",\"label\":\"A\",\"type\":\"foundation.hydraulic.hydraulic\"}],\"Right\":[{\"id\":\"B\",\"label\":\"B\",\"type\":\"foundation.hydraulic.hydraulic\"}],\"Top\":[]}"
  Hydraulic Flow Rate Sensor : fl_lib/Hydraulic/Hydraulic Sensors/Hydraulic Flow Rate Sensor
  Hydraulic Fluid : sh_lib/Hydraulic Utilities/Hydraulic Fluid  SelFluid=22  SysTemp=60  TrapAir=0.005  ViscDerFactor=1  range_error=2
  Hydraulic Reference : fl_lib/Hydraulic/Hydraulic Elements/Hydraulic Reference
  Ideal Angular Velocity Source1 : fl_lib/Mechanical/Mechanical Sources/Ideal Angular Velocity Source
  Mechanical Rotational Reference1 : fl_lib/Mechanical/Rotational Elements/Mechanical Rotational Reference
  PS Constant : fl_lib/Physical Signals/Sources/PS Constant  constant=1
  PS-Simulink Converter : nesl_utility/PS-Simulink Converter  PhysicalDomain=network_engine_domain  SubClassName=ps_output  LeftPortType=input  RightPortType=output  PseudoPeriodic=off  Frequencies=[]  VectorFormat=inherit  Unit=inherit  AffineConversion=off
  Pressure Relief Valve : sh_lib/Valves/Pressure Control Valves/Pressure Relief Valve  valve_area_spec=1  p_diff_TLU=[30.15e5 : 15e3 : 31.35e5] Pa  area_TLU=[1 : 1 : 9] .* 1e-5 m^2  area_max=1e-4 m^2  pres_set=50e5 Pa  reg_range=5e5 Pa  C_d=0.7  A_leak=1e-12 m^2  lam_spec=1  B_lam=0.999  Re_cr=12  dynamic=0  tau=0.1 s  area_init=1e-12 m^2
      settings: InternalSimscapePortConfiguration="{\"Bottom\":[],\"Left\":[{\"id\":\"A\",\"label\":\"A\",\"type\":\"foundation.hydraulic.hydraulic\"}],\"Right\":[{\"id\":\"B\",\"label\":\"B\",\"type\":\"foundation.hydraulic.hydraulic\"}],\"Top\":[]}"
  Rate 100Hz1 : RateTransition  OutPortSampleTimeMultiple=2  OutPortSampleTime=0.2
  Rate 100Hz2 : RateTransition  InitialCondition=1  OutPortSampleTimeMultiple=2  OutPortSampleTime=0.2
  Simulink-PS Converter : nesl_utility/Simulink-PS Converter  PhysicalDomain=network_engine_domain  SubClassName=ps_input  LeftPortType=input  RightPortType=output  PseudoPeriodic=off  Frequencies=[]  NoiseDistribution=none  NoiseParameters=[]  Unit=1  AffineConversion=off  FilteringAndDerivatives=provide  SimscapeFilterOrder=1  InputFilterTimeConstant=0.001  UdotUserProvided=0
  Simulink-PS Converter1 : nesl_utility/Simulink-PS Converter  PhysicalDomain=network_engine_domain  SubClassName=ps_input  LeftPortType=input  RightPortType=output  PseudoPeriodic=off  Frequencies=[]  NoiseDistribution=none  NoiseParameters=[]  Unit=1  AffineConversion=off  FilteringAndDerivatives=provide  SimscapeFilterOrder=1  InputFilterTimeConstant=0.001  UdotUserProvided=0
  Solver Configuration : nesl_utility/Solver Configuration  PhysicalDomain=network_engine_domain  SubClassName=solver  LeftPortType=input  RightPortType=generic  Tones=[]  Harmonics=[]  SimulateNoise=off  Profile=off  UseLocalSampling=off  EnableSwitchedLinearOptims=on  FrequencyDomain=off  UseCCode=off  RelTol=0.001  AbsTol=0.001  MinStep=1e-09  ToWorkspace=off  RevertToSquareIcSolve=off  NumHomotopyIterations=100  PhasorMode=off  PhasorModeNumHarmonics=1  ConsistencySolver=NEWTON_XTOL_AFTER_FTOL  IndexReductionMethod=DerivativeReplacement  DoDC=off  ResidualTolerance=1e-09  ConsistencyTolSource=GLOBAL  ConsistencyAbsTol=0.001  ConsistencyRelTol=0.001  ConsistencyTolFactor=0.001  UseLocalSolver=off  LocalSolverChoice=NE_BACKWARD_EULER_ADVANCER  ResolveIndetEquations=on  FunctionEvalNumThread=1  LocalSolverSampleTime=0.001  DoFixedCost=off  MaxNonlinIter=3  MaxModeIter=2  ComputeImpulses=off  ImpulseIterations=2  LinearAlgebra=auto  LinearAlgebraNumThread=0  EquationFormulation=NE_TIME_EF  DelaysMemoryBudget=1024  AutomaticFiltering=on  FilteringTimeConstant=0.001  PartitionStorageMethod=AS_NEEDED  PartitionMemoryBudget=1024  PartitionMethod=ROBUST
  Variable-Displacement Pump1 : sh_lib/Pumps and Motors/Variable-Displacement Pump  mdl_type=1  stroke_max=0.005 m  D_max=30 cm^3/rev  cntrl_mem_tab=[-.0075, -.0025, 0, .0025, .0075] m  displ_tab=[-30, -19, 0, 19, 30] cm^3/rev  interp_method=1  extrap_method=1  loss_spec=1  w_nominal=188 rad/s  pr_nominal=100e5 Pa  visc_nominal=18 cSt  dens_nominal=900 kg/m^3  efficiency_vol=0.92  no_load_torque=0.05 N*m  torque_pressure_coeff=0.6e-6 N*m/Pa  p_diff_eff_TLU=[100000, 1000000, 2000000] Pa  omega_eff_TLU=[25, 50, 100, 200, 300, 400] rad/s  displacement_eff_TLU=[-30, -19, 19, 30] cm^3/rev  vol_eff_TLU=repmat([.816, .908, .954, .977, .981, .984; .325, .663, .831, .916, .925, .946; .137, .568, .78, .892, .893, .91], 1, 1, 4)  mech_eff_TLU=repmat([.996, .996, .996, .996, .996, .996; .988, .989, .989, .989, .989, .99; .981, .981, .982, .982, .983, .984], 1, 1, 4)  p_diff_loss_TLU=[100000, 1000000, 2000000] Pa  omega_loss_TLU=[25, 50, 100, 200, 300, 400] rad/s  displacement_loss_TLU=[-30, -19, 19, 30] cm^3/rev  vol_loss_TLU=repmat([.023, .023, .023, .023, .0285, .032; .0844, .0842, .0845, .084, .1125, .108; .1079, .108, .11, .108, .1605, .18] * 1e-3, 1, 1, 4) m^3/s  mech_loss_TLU=repmat([.002, .002, .002, .002, .002, .002; .0607, .0556, .0556, .0556, .0556, .0505; .1937, .1937, .1833, .1833, .1729, .1626], 1, 1, 4) N*m  pressure_threshold=1e5 Pa  omega_threshold=10 rad/s  displacement_threshold=0.5 cm^3/rev  octant_check=0  pressure_check=0  min_valid_pressure=0 Pa  vol_eff_min=1e-3  vol_eff_max=1  mech_eff_min=1e-3  mech_eff_max=1
      settings: InternalSimscapePortConfiguration="{\"Bottom\":[],\"Left\":[{\"id\":\"C\",\"label\":\"C\",\"type\":\"input\"},{\"id\":\"S\",\"label\":\"S\",\"type\":\"foundation.mechanical.rotational.rotational\"}],\"Right\":[{\"id\":\"P\",\"label\":\"P\",\"type\":\"foundation.hydraulic.hydraulic\"},{\"id\":\"T\",\"label\":\"T\",\"type\":\"foundation.hydraulic.hydraulic\"}],\"Top\":[]}"
  FMV flow rate [%] : Outport
  Wf : Outport  Port=2
  Wf true : Outport  Port=3
  wires:
  100%- 0.044 kg/s/1 -> Divide/2
  SOV signal/1 -> Simulink-PS Converter1/1
  PS-Simulink Converter/1 -> Rate 100Hz1/1, Wf/1, Divide/1  "Wf"
  Rate 100Hz1/1 -> Wf true/1
  Divide/1 -> Rate 100Hz2/1  "w"
  signal to FMV/1 -> Simulink-PS Converter/1
  Rate 100Hz2/1 -> FMV flow rate [%]/1
  connections:
  Pressure Relief Valve/RConn1 -- Hydraulic Flow Rate Sensor/RConn2 -- Hydraulic Fluid/RConn1 -- Solver Configuration/RConn1 -- Hydraulic Reference/LConn1 -- Pressure Relief Valve/LConn1 -- Variable-Displacement Pump1/RConn2
  Simulink-PS Converter/RConn1 -- Ideal Angular Velocity Source1/RConn1
  Ideal Angular Velocity Source1/RConn2 -- Mechanical Rotational Reference1/LConn1
  Variable-Displacement Pump1/LConn2 -- Ideal Angular Velocity Source1/LConn1
  Hydraulic Flow Rate Sensor/RConn3 -- PS-Simulink Converter/LConn1
  Variable-Displacement Pump1/LConn1 -- PS Constant/RConn1
  Simulink-PS Converter1/RConn1 -- Gate Valve/LConn1
  Variable-Displacement Pump1/RConn1 -- Gate Valve/LConn2
  Hydraulic Flow Rate Sensor/LConn1 -- Gate Valve/RConn1

== system simulation model/ECU /FMV sensor ==
  FMVact pos : Inport
  Add2 : Sum
  Product2 : Product
  Rate 100Hz1 : RateTransition  OutPortSampleTimeMultiple=2  OutPortSampleTime=0.01
  normal noise1 : UniformRandomNumber  Seed=1  SampleTime=0.1
  FMVact sens : Outport
  wires:
  Rate 100Hz1/1 -> Add2/1, Product2/1
  Add2/1 -> FMVact sens/1
  FMVact pos/1 -> Rate 100Hz1/1
  normal noise1/1 -> Product2/2
  Product2/1 -> Add2/2

== system simulation model/ECU /Ng sensor ==
  Ng : Inport
  Add : Sum
  Add1 : Sum
  Bus Creator : BusCreator  Inputs=2
  Normal Noise : RandomNumber  Variance=((0.017)^2)*pi/2  Seed=10  SampleTime=0.01
  Normal Noise1 : RandomNumber  Variance=((0.017)^2)*pi/2  Seed=11  SampleTime=0.01
  Product : Product
  Product1 : Product
  Rate 100Hz : RateTransition  OutPortSampleTimeMultiple=2  OutPortSampleTime=0.01
  Ngsen : Outport
  wires:
  Product/1 -> Add/2
  Product1/1 -> Add1/2
  Normal Noise1/1 -> Product1/2
  Rate 100Hz/1 -> Add/1, Product/1, Add1/1, Product1/1
  Ng/1 -> Rate 100Hz/1
  Add1/1 -> Bus Creator/2
  Add/1 -> Bus Creator/1
  Bus Creator/1 -> Ngsen/1
  Normal Noise/1 -> Product/2

== system simulation model/ECU /Ng speed limiters ==
  Ng_sen : Inport
  Add : Sum
  Constant : Constant  Value=-1
  Constant1 : Constant
  Demux : Demux  Outputs=2
  Gain : Gain  Gain=0.5
  Safe switch : Subsystem
  Switch : Switch  Criteria=u2 > Threshold  Threshold=Ng_safe  SaturateOnIntegerOverflow=off  InputSameDT=off
  Ng to SOV : Outport
  wires:
  Constant/1 -> Switch/3
  Constant1/1 -> Switch/1
  Ng_sen/1 -> Demux/1
  Demux/1 -> Add/1
  Demux/2 -> Add/2
  Gain/1 -> Switch/2
  Add/1 -> Gain/1
  Switch/1 -> Safe switch/1(In1)
  Safe switch/1(Out1) -> Ng to SOV/1

== system simulation model/ECU /No sensor ==
  Np : Inport
  Add1 : Sum
  Add2 : Sum
  Bus Creator : BusCreator  Inputs=2
  Normal Noise1 : RandomNumber  Variance=((0.017)^2)*pi/2  Seed=16  SampleTime=0.01
  Normal Noise2 : RandomNumber  Variance=((0.017)^2)*pi/2  Seed=18  SampleTime=0.01
  Product1 : Product
  Product2 : Product
  Rate 100Hz1 : RateTransition  OutPortSampleTimeMultiple=2  OutPortSampleTime=0.01
  Nosen : Outport
  wires:
  Np/1 -> Rate 100Hz1/1
  Normal Noise2/1 -> Product2/2
  Rate 100Hz1/1 -> Add2/1, Product2/1, Add1/1, Product1/1
  Add2/1 -> Bus Creator/2
  Add1/1 -> Bus Creator/1
  Bus Creator/1 -> Nosen/1
  Normal Noise1/1 -> Product1/2
  Product1/1 -> Add1/2
  Product2/1 -> Add2/2

== system simulation model/ECU /No speed limiters ==
  Nosen : Inport
  Add : Sum
  Constant : Constant  Value=-1
  Constant1 : Constant
  Demux : Demux  Outputs=2
  Gain : Gain  Gain=0.5
  No_performance : Constant  Value=No_perf
  Safe switch : Subsystem
  Subtract : Sum  Inputs=+-
  Switch : Switch  Criteria=u2 > Threshold  Threshold=No_safe  SaturateOnIntegerOverflow=off  InputSameDT=off
  No to PCV : Outport
  No to FBV : Outport  Port=2
  wires:
  Add/1 -> Gain/1
  Nosen/1 -> Demux/1
  Demux/1 -> Add/1
  Demux/2 -> Add/2
  Constant/1 -> Switch/3
  Constant1/1 -> Switch/1
  Gain/1 -> Subtract/1, Switch/2
  No_performance/1 -> Subtract/2
  Subtract/1 -> No to PCV/1
  Switch/1 -> Safe switch/1(In1)
  Safe switch/1(No to FBV) -> No to FBV/1

== system simulation model/ECU /Np sensor ==
  Np : Inport
  Add : Sum
  Add1 : Sum
  Bus Creator : BusCreator  Inputs=2
  Normal Noise1 : RandomNumber  Variance=((0.017)^2)*pi/2  Seed=13  SampleTime=0.01
  Normal Noise2 : RandomNumber  Variance=((0.017)^2)*pi/2  Seed=14  SampleTime=0.01
  Product : Product
  Product1 : Product
  Rate 100Hz : RateTransition  OutPortSampleTimeMultiple=2  OutPortSampleTime=0.01
  Npsen : Outport
  wires:
  Normal Noise1/1 -> Product/2
  Product/1 -> Add/2
  Np/1 -> Rate 100Hz/1
  Normal Noise2/1 -> Product1/2
  Product1/1 -> Add1/2
  Rate 100Hz/1 -> Add/1, Product/1, Add1/1, Product1/1
  Add1/1 -> Bus Creator/2
  Add/1 -> Bus Creator/1
  Bus Creator/1 -> Npsen/1

== system simulation model/ECU /Np speed limiters ==
  Npsen : Inport
  Add : Sum
  Constant : Constant  Value=-1
  Constant1 : Constant
  Demux : Demux  Outputs=2
  Gain : Gain  Gain=0.5
  Safe switch : Subsystem
  Switch : Switch  Criteria=u2 > Threshold  Threshold=Np_safe  SaturateOnIntegerOverflow=off  InputSameDT=off
  Np to SOV : Outport
  wires:
  Switch/1 -> Safe switch/1(In1)
  Constant1/1 -> Switch/1
  Constant/1 -> Switch/3
  Gain/1 -> Switch/2
  Demux/2 -> Add/2
  Npsen/1 -> Demux/1
  Add/1 -> Gain/1
  Demux/1 -> Add/1
  Safe switch/1(Np to SOV) -> Np to SOV/1

== system simulation model/ECU /P0 sensor ==
  P0 : Inport
  Add : Sum
  Add1 : Sum
  Bus Creator : BusCreator  Inputs=2
  Delay : Delay  DelayLength=10  InitialCondition=1  SampleTime=0.001
  Normal Noise : RandomNumber  Variance=((0.005)^2)*pi/2  Seed=31  SampleTime=0.01
  Normal Noise1 : RandomNumber  Variance=((0.005)^2)*pi/2  Seed=33  SampleTime=0.01
  Product : Product
  Product1 : Product
  Rate 100Hz : RateTransition  OutPortSampleTimeMultiple=2  OutPortSampleTime=0.01
  P0sen : Outport
  wires:
  P0/1 -> Delay/1
  Normal Noise1/1 -> Product1/2
  Normal Noise/1 -> Product/2
  Add1/1 -> Bus Creator/2
  Bus Creator/1 -> P0sen/1
  Product1/1 -> Add1/2
  Product/1 -> Add/2
  Rate 100Hz/1 -> Add1/1, Product1/1, Add/1, Product/1
  Add/1 -> Bus Creator/1
  Delay/1 -> Rate 100Hz/1

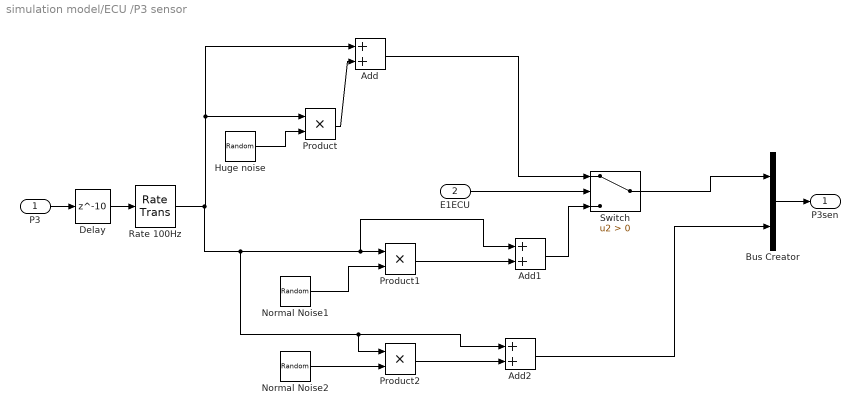
== system simulation model/ECU /P3 sensor ==
  P3 : Inport
  E1ECU : Inport  Port=2
  Add : Sum
  Add1 : Sum
  Add2 : Sum
  Bus Creator : BusCreator  Inputs=2
  Delay : Delay  DelayLength=10  InitialCondition=1  SampleTime=0.001
  Huge noise : RandomNumber  Variance=((0.03)^2)*pi/2  Seed=1  SampleTime=0.01
  Normal Noise1 : RandomNumber  Variance=((0.005)^2)*pi/2  Seed=2  SampleTime=0.01
  Normal Noise2 : RandomNumber  Variance=((0.005)^2)*pi/2  Seed=4  SampleTime=0.01
  Product : Product
  Product1 : Product
  Product2 : Product
  Rate 100Hz : RateTransition  OutPortSampleTimeMultiple=2  OutPortSampleTime=0.01
  Switch : Switch  Criteria=u2 > Threshold  SaturateOnIntegerOverflow=off  InputSameDT=off
  P3sen : Outport
  wires:
  Bus Creator/1 -> P3sen/1
  P3/1 -> Delay/1
  Normal Noise2/1 -> Product2/2
  Add/1 -> Switch/1
  Huge noise/1 -> Product/2
  Add1/1 -> Switch/3
  Product/1 -> Add/2
  Product2/1 -> Add2/2
  Rate 100Hz/1 -> Add2/1, Product2/1, Add1/1, Product1/1, Product/1, Add/1
  Add2/1 -> Bus Creator/2
  Normal Noise1/1 -> Product1/2
  Switch/1 -> Bus Creator/1
  E1ECU/1 -> Switch/2
  Product1/1 -> Add1/2
  Delay/1 -> Rate 100Hz/1

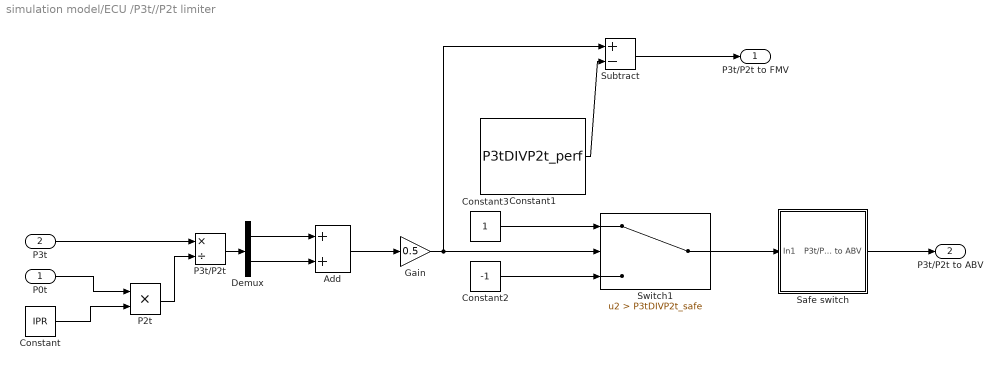
== system simulation model/ECU /P3t//P2t limiter ==
  P0t : Inport
  P3t : Inport  Port=2
  Add : Sum
  Constant : Constant  Value=IPR
  Constant1 : Constant  Value=P3tDIVP2t_perf
  Constant2 : Constant  Value=-1
  Constant3 : Constant
  Demux : Demux  Outputs=2
  Gain : Gain  Gain=0.5
  P2t : Product
  P3t/P2t : Product  Inputs=*/
  Safe switch : Subsystem
  Subtract : Sum  Inputs=+-
  Switch1 : Switch  Criteria=u2 > Threshold  Threshold=P3tDIVP2t_safe  SaturateOnIntegerOverflow=off  InputSameDT=off
  P3t/P2t to FMV : Outport
  P3t/P2t to ABV : Outport  Port=2
  wires:
  Subtract/1 -> P3t/P2t to FMV/1
  P3t/1 -> P3t/P2t/1
  Constant1/1 -> Subtract/2
  Gain/1 -> Switch1/2, Subtract/1
  Constant2/1 -> Switch1/3
  Switch1/1 -> Safe switch/1(In1)
  Constant3/1 -> Switch1/1
  Demux/2 -> Add/2
  Demux/1 -> Add/1
  Add/1 -> Gain/1
  P3t/P2t/1 -> Demux/1
  Safe switch/1(P3t/P2t to ABV) -> P3t/P2t to ABV/1
  P0t/1 -> P2t/1
  P2t/1 -> P3t/P2t/2
  Constant/1 -> P2t/2

== system simulation model/ECU /PCV controller ==
  Signal to FBV : Inport
  No to PCV : Inport  Port=2
  Constant : Constant  Value=-0.005
  PID Controller : slpidlib/PID Controller  Controller=PI  Form=Parallel  TimeDomain=Discrete-time  UseExternalTs=off  SampleTime=0.1  IntegratorMethod=Forward Euler  FilterMethod=Forward Euler  ControllerParametersSource=internal  P=-0.01  I=1*10^-6  UseKiTs=off  D=0  N=100  UseFilter=on  TunerSelectOption=Transfer Function Based (PID Tuner App)  InitialConditionSource=internal  InitialConditionForIntegrator=0  InitialConditionForFilter=0  DifferentiatorICPrevScaledInput=0  ExternalReset=none  TrackingMode=off  Kt=1  LimitOutput=on  SatLimitsSource=internal  UpperSaturationLimit=20  LowerSaturationLimit=-20  LinearizeAsGain=on  AntiWindupMode=none  Kb=1  LimitIntegrator=on  UpperIntegratorSaturationLimit=20  LowerIntegratorSaturationLimit=-20  POutMin=[]  POutMax=[]  IOutMin=[]  IOutMax=[]  DOutMin=[]  DOutMax=[]  NOutMin=[]  NOutMax=[]  SumOutMin=[]  SumOutMax=[]  SaturationOutMin=[]  SaturationOutMax=[]  PParamMin=[]  PParamMax=[]  IParamMin=[]  IParamMax=[]  DParamMin=[]  DParamMax=[]  NParamMin=[]  NParamMax=[]  KbParamMin=[]  KbParamMax=[]  KtParamMin=[]  KtParamMax=[]  KbOutMin=[]  KbOutMax=[]  KtOutMin=[]  KtOutMax=[]  IntegratorOutMin=[]  IntegratorOutMax=[]  FilterOutMin=[]  FilterOutMax=[]  SumI1OutMin=[]  SumI1OutMax=[]  SumI2OutMin=[]  SumI2OutMax=[]  SumI3OutMin=[]  SumI3OutMax=[]  SumI4OutMin=[]  SumI4OutMax=[]  SumDOutMin=[]  SumDOutMax=[]  DifferentiatorOutMin=[]  DifferentiatorOutMax=[]  FilterDiffOutCoefMin=[]  FilterDiffOutCoefMax=[]  ReciprocalOutMin=[]  ReciprocalOutMax=[]  SumDenOutMin=[]  SumDenOutMax=[]  SumNumOutMin=[]  SumNumOutMax=[]  DivideOutMin=[]  DivideOutMax=[]  UdiffTsProdOutMin=[]  UdiffTsProdOutMax=[]  NTsProdOutMin=[]  NTsProdOutMax=[]  UintegralTsProdOutMin=[]  UintegralTsProdOutMax=[]  UngainTsProdOutMin=[]  UngainTsProdOutMax=[]  ClampingZeroOutDataTypeStr=Inherit: Inherit via back propagation  ClampingZeroOutMin=[]  ClampingZeroOutMax=[]  FilterDenConstantOutDataTypeStr=Inherit: Inherit via back propagation  FilterDenConstantOutMin=[]  FilterDenConstantOutMax=[]  PCopyOutDataTypeStr=Inherit: Inherit via back propagation  PCopyOutMin=[]  PCopyOutMax=[]  NCopyOutDataTypeStr=Inherit: Inherit via back propagation  NCopyOutMin=[]  NCopyOutMax=[]  IntegratorContinuousStateAttributes=''  IntegratorStateMustResolveToSignalObject=off  IntegratorRTWStateStorageClass=Auto  FilterContinuousStateAttributes=''  FilterStateMustResolveToSignalObject=off  FilterRTWStateStorageClass=Auto  ParallelPVariant=InternalParameters  IdealPVariant=Disabled  IVariant=InternalParameters  DVariant=Disabled  IntegratorVariant=Discrete  SatVariant=Enabled  AWVariant=Passthrough  PCopyVariant=Disabled  TRVariant=Disabled  FdbkBlocksVariant=Forward  IdealPFdbkVariant=Disabled  SatFdbkVariant=Disabled  DerivativeFilterVariant=Disabled  NVariant=Disabled  NCopyVariant=Disabled_SignalSpec  FilterICVariant=Disabled  IntegratorICVariant=InternalICs  ExternalResetVariant=Disabled  TRSumVariant=Passthrough  SumFdbkVariant=Disabled  SumVariant=Sum_PI  TsampFilterVariant=InternalTs  TsampNgainVariant=Passthrough  TsampIntegralVariant=Passthrough  ExternalSaturationOutDataTypeStr=Inherit: Same as second input
  Switch : Switch  Criteria=u2 > Threshold  SaturateOnIntegerOverflow=off  InputSameDT=off
  PCV signal : Outport
  FBV signal : Outport  Port=2
  wires:
  No to PCV/1 -> PID Controller/1
  PID Controller/1 -> Switch/1
  Signal to FBV/1 -> FBV signal/1, Switch/2
  Switch/1 -> PCV signal/1
  Constant/1 -> Switch/3
